simulink model "controller"  (R2020a)
settings: Solver=FixedStepDiscrete  StartTime=0.0  StopTime=10.0  FixedStep=0.01  MaxStep=0.01  RelTol=1e-3
undefined symbols (not defined in the file): DiscIntNeverNeededParam, PC_IST_den, PC_IST_num
libraries: simulink x10, dspsigattribs x1, dspfdesign x1
Description:
  | Ventilator Controller
settings Model: Creator=upattacini  LastModifiedBy=upattacini
settings SolverCC: MaxConsecutiveMinStep=10
settings DataIOCC: SaveOutput=off  SignalLogging=off  DSMLogging=off  SaveTime=off  ReturnWorkspaceOutputs=off
settings OptimizationCC: DefaultUnderspecifiedDataType=single  StrengthReduction=on  ZeroExternalMemoryAtStartup=off  ZeroInternalMemoryAtStartup=off  OptimizeBlockOrder=speed  OptimizationPriority=Speed  OptimizationCustomize=off  MultiThreadedLoops=on  EfficientTunableParamExpr=on
settings DebuggingCC: ParameterTunabilityLossMsg=error
settings SFSimCC: MATLABDynamicMemAlloc=off
settings RTWCC: SystemTargetFile=ert.tlc  GenCodeOnly=on  PackageGeneratedCodeAndArtifacts=on  PackageName=controller  TemplateMakefile=ert_default_tmf  TargetLang=C++
settings CodeAppCC: ForceParamTrailComments=on  IgnoreCustomStorageClasses=off  OperatorAnnotations=on  SimulinkDataObjDesc=on  SFDataObjDesc=on  InsertBlockDesc=on
settings ERTTargetCC: TargetLangStandard=C++03 (ISO)  GenerateSampleERTMain=on  MultiInstanceERTCode=on  CodeInterfacePackaging=C++ class  RootIOFormat=Structure reference  ERTCustomFileTemplate=example_file_process.tlc

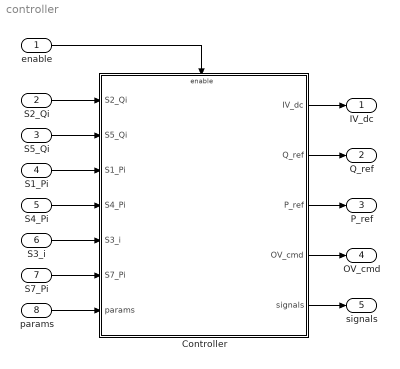
== system controller ==
  enable : Inport  OutDataTypeStr=boolean
  S2_Qi : Inport  Port=2  OutDataTypeStr=single
  S5_Qi : Inport  Port=3  OutDataTypeStr=single
  S1_Pi : Inport  Port=4  OutDataTypeStr=single
  S4_Pi : Inport  Port=5  OutDataTypeStr=single
  S3_i : Inport  Port=6  OutDataTypeStr=single  PortDimensions=2
  S7_Pi : Inport  Port=7  OutDataTypeStr=single
  params : Inport  Port=8  OutDataTypeStr=single  PortDimensions=3
  Controller : Subsystem  Tag=PublishSubsystem  mask(Controller){control_mode=IDLE, tidal_volume=0.65, PIP=25, PIP_step_perc=75, PIP_rise_perc=70, respiratory_rate=10, IE_ratio=1/2, HSC_cutoff=25, recovery_thres=1, VC_P=0.2, VC_I=10, VC_P_rec=0.1, VC_I_rec=5, PC_FFW=30, PC_P=1, PC_I=40, PC_FFW_rec=30, PC_P_rec=0.05, PC_I_rec=10, enable_trigger=off, pressure_thres=3, flowby_target=3}
      mask prompts: control_mode "Control Mode"; tidal_volume "Tidal Volume (L)"; PIP "PIP (cmH2O)"; PIP_step_perc "PIP Step Percentage (%)"; PIP_rise_perc "PIP Rising Percentage (%)"; respiratory_rate "Respiratory Rate (breaths/min)"; IE_ratio "Inspiration to Expiration Ratio"; HSC_cutoff "HSC Cutoff Frequency (Hz)"; recovery_thres "Threshold (bar)"; VC_P "Proportional (%FS/SLPM)"; VC_I "Integral (%FS/(SLPM*s))"; VC_P_rec "Proportional (%FS/SLPM)"; VC_I_rec "Integral (%FS/(SLPM*s))"; PC_FFW "Feed-Forward (%FS)"; PC_P "Proportional (%FS/cmH2O)"; PC_I "Integral (%FS/(cmH2O*s))"; PC_FFW_rec "Feed-Forward (%FS)"; PC_P_rec "Proportional (%FS/cmH2O)"; PC_I_rec "Integral (%FS/(cmH2O*s))"; enable_trigger "Enable Triggering"; pressure_thres "Pressure Threshold (cmH2O)"; flowby_target "Target Flow (L/min)"
      mask help: The controller generates the input signals that controls the inspiratory flow and expiratory valve.
      mask init:
      | Ts = eval(get_param(gcs, 'FixedStep'));
      mask TypeOptions control_mode: IDLE | CPAP | VCV | PRVC
      mask Callback control_mode:
      | numparams = Simulink.Mask.get(gcb).numParameters;
      | enable = cell(1, numparams);
      | enable(:) = {'on'};
      | 
      | control_mode = get_param(gcb, 'control_mode');
      | if strcmpi(control_mode, 'CPAP')
      |     enable{2} = 'off';
      |     enable(6:7) = {'off'};
      |     enable(10:13) = {'off'};
      | elseif strcmpi(control_mode, 'VCV')
      |     enable(3:5) = {'off'};
      |     enable(14:19) = {'off'};
      | elseif strcmpi(control_mode, 'PRVC')
      |     enable{2} = 'off';
      |     enable(10:13) = {'off'};
      | else
      |     enable(2:end) = {'off'};
      |     enable{8} = 'on';
      | end
      | if strcmpi(control_mode, 'CPAP')
      |     enable(end-2:end) = {'off'};
      | end
      | set_param(gcb, 'MaskEnables', enable);
      mask DialogControl Container2 Prompt: Medical Parameters
      mask DialogControl Container3 Prompt: Controller Parameters
      mask DialogControl Container4 Prompt: Filtering
      mask DialogControl Container5 Prompt: Gain Scheduling
      mask DialogControl Container6 Prompt: Volume Control Ventilation
      mask DialogControl Container7 Prompt: Standard Operations
      mask DialogControl Container8 Prompt: Recovery Operations
      mask DialogControl Container9 Prompt: Pressure Regulated Volume Control
      mask DialogControl Container10 Prompt: Standard Operations
      mask DialogControl Container11 Prompt: Recovery Operations
      mask DialogControl Container12 Prompt: Advanced Options
      mask DialogControl Container13 Prompt: Assisted Ventilation
      mask DialogControl Container14 Prompt: Flow-by
  IV_dc : Outport
  Q_ref : Outport  Port=2
  P_ref : Outport  Port=3
  OV_cmd : Outport  Port=4
  signals : Outport  Port=5
  wires:
  S2_Qi/1 -> Controller/1(S2_Qi)
  Controller/1(IV_dc) -> IV_dc/1
  Controller/2(Q_ref) -> Q_ref/1
  Controller/4(OV_cmd) -> OV_cmd/1
  S1_Pi/1 -> Controller/3(S1_Pi)
  Controller/3(P_ref) -> P_ref/1
  Controller/5(signals) -> signals/1
  enable/1 -> Controller/Enable
  S5_Qi/1 -> Controller/2(S5_Qi)
  S4_Pi/1 -> Controller/4(S4_Pi)
  params/1 -> Controller/7(params)
  S3_i/1 -> Controller/5(S3_i)
  S7_Pi/1 -> Controller/6(S7_Pi)

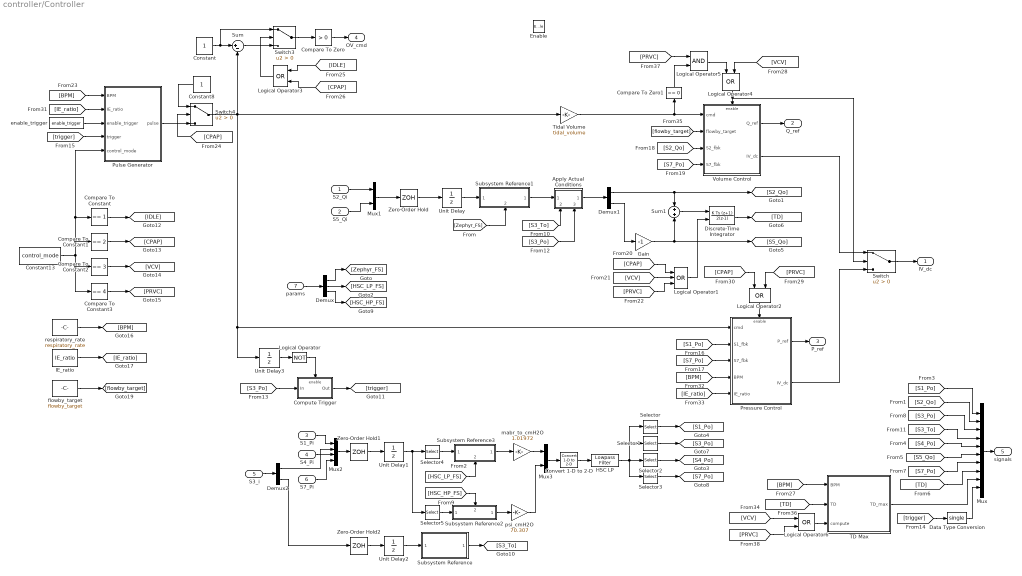
== system controller/Controller ==
  S2_Qi : Inport
  S5_Qi : Inport  Port=2
  S1_Pi : Inport  Port=3
  S4_Pi : Inport  Port=4
  S3_i : Inport  Port=5
  S7_Pi : Inport  Port=6
  params : Inport  Port=7
  Enable : EnablePort  StatesWhenEnabling=reset
  Apply Actual Conditions : Subsystem  ReferencedSubsystem=apply_actual_conditions
      settings: PortSchema="{\"entries\":[{\"content\":{\"sides\":[{\"content\":{\"connectorIds\":[\"In1\"]},\"type\":\"ConnectorPlacement.EquallySpacedRectSide\",\"uuid\":\"3b4e15f5-ec7a-455d-a112-e063b421ee9f\"},{\"content\":{\"connectorIds\":[\"Out1\"],\"side\":\"RIGHT\"},\"type\":\"ConnectorPlacement.EquallySpacedRectSide\",\"uuid\":\"595b3fd5-6603-4191-b183-4edf5336d9a2\"},{\"content\":{\"connectorIds\":[],\"side\":\"TOP\"},\"type\":\"ConnectorPlacement.EquallySpacedRectSide\",\"uuid\":\"7211f4ea-7225-4536-b1e6-5aea95971c19\"},{\"content\":{\"connectorIds\":[\"In2\",\"In3\"],\"side\":\"BOTTOM\"},\"type\":\"ConnectorPlacement.EquallySpacedRectSide\",\"uuid\":\"c060314b-2654-4a54-a68c-60767f6efbb5\"}]},\"type\":\"ConnectorPlacement.EquallySpacedConnector\",\"uuid\":\"0e2934c3-16fd-4aed-85e0-c12757e58969\"}],\"packageUris\":[\"http://schema.mathworks.com/mf0/Connector/19700101\"],\"version\":\"1.0\"}"
  Compare To Constant : simulink/Logic and Bit Operations/Compare To Constant  relop===  const=1  OutDataTypeStr=boolean
  Compare To Constant1 : simulink/Logic and Bit Operations/Compare To Constant  relop===  const=2  OutDataTypeStr=boolean
  Compare To Constant2 : simulink/Logic and Bit Operations/Compare To Constant  relop===  const=3  OutDataTypeStr=boolean
  Compare To Constant3 : simulink/Logic and Bit Operations/Compare To Constant  relop===  const=4  OutDataTypeStr=boolean
  Compare To Zero : simulink/Logic and Bit Operations/Compare To Zero  relop=>  OutDataTypeStr=boolean
  Compare To Zero1 : simulink/Logic and Bit Operations/Compare To Zero  relop===  OutDataTypeStr=boolean
  Compute Trigger : Subsystem
  Constant : Constant  OutDataTypeStr=single
  Constant13 : Constant  Value=control_mode  OutDataTypeStr=uint8
  Constant8 : Constant  OutDataTypeStr=single
  Convert 1-D to 2-D : dspsigattribs/Convert 1-D to 2-D  M=1  N=4  frameBasedOut=off
      settings: SourceProductBaseCode=DS
  Data Type Conversion : DataTypeConversion  OutDataTypeStr=single
  Demux : Demux  Outputs=3
  Demux1 : Demux  Outputs=2
  Demux2 : Demux  Outputs=2
  Discrete-Time Integrator : DiscreteIntegrator  IntegratorMethod=Integration: Trapezoidal  gainval=1/60  ExternalReset=rising  SampleTime=-1  ICPrevOutput=DiscIntNeverNeededParam  ICPrevScaledInput=DiscIntNeverNeededParam
  Gain : Gain  Gain=-1
  HSC LP : dspfdesign/Lowpass Filter  FilterType=IIR  DesignForMinimumOrder=off  FilterOrder=3  PassbandFrequency=HSC_cutoff  StopbandFrequency=12e3  PassbandRipple=0.5  StopbandAttenuation=30  InheritSampleRate=on  SampleRate=44100  SimulateUsing=Code generation  roundingMode=Floor  coeffsDataTypeStr=fixdt(1,16)
  IE_ratio : Constant  Value=IE_ratio  OutDataTypeStr=single
  Logical Operator : Logic  Operator=NOT  AllPortsSameDT=off  OutDataTypeStr=boolean
  Logical Operator1 : Logic  Operator=OR  Inputs=3  AllPortsSameDT=off  OutDataTypeStr=boolean
  Logical Operator{2..4,6} (4 alike) : Logic  Operator=OR  AllPortsSameDT=off  OutDataTypeStr=boolean
  Logical Operator5 : Logic  AllPortsSameDT=off  OutDataTypeStr=boolean
  Mux : Mux  Inputs=10
  Mux1 : Mux  Inputs=2
  Mux2 : Mux
  Mux3 : Mux  Inputs=2
  Pressure Control : Subsystem
  Pulse Generator : Stateflow chart  TreatAsAtomicUnit=on
      settings: PortSchema="{\"entries\":[{\"content\":{\"sides\":[{\"content\":{\"connectorIds\":[\"In1\",\"In2\",\"In4\",\"In5\",\"In3\"]},\"type\":\"ConnectorPlacement.EquallySpacedRectSide\",\"uuid\":\"cac98c0d-34b3-4e58-8046-b8c4efc2c89e\"},{\"content\":{\"connectorIds\":[\"Out1\"],\"side\":\"RIGHT\"},\"type\":\"ConnectorPlacement.EquallySpacedRectSide\",\"uuid\":\"54f456d4-4e16-46b8-85c9-ac589a430e9a\"},{\"content\":{\"connectorIds\":[],\"side\":\"TOP\"},\"type\":\"ConnectorPlacement.EquallySpacedRectSide\",\"uuid\":\"89fc85cb-8402-4155-a34e-39605e1a4b07\"}]},\"type\":\"ConnectorPlacement.EquallySpacedConnector\",\"uuid\":\"7c549002-3361-42b3-b309-390e5b6446c3\"}],\"packageUris\":[\"http://schema.mathworks.com/mf0/Connector/19700101\"],\"version\":\"1.0\"}"
  Selector : Selector  InputPortWidth=4  IndexOptions=Index vector (dialog)  Indices=1  OutputSizes=1
  Selector1 : Selector  InputPortWidth=4  IndexOptions=Index vector (dialog)  Indices=2  OutputSizes=1
  Selector2 : Selector  InputPortWidth=4  IndexOptions=Index vector (dialog)  Indices=3  OutputSizes=1
  Selector3 : Selector  InputPortWidth=4  IndexOptions=Index vector (dialog)  Indices=4  OutputSizes=1
  Selector4 : Selector  InputPortWidth=4  IndexOptions=Index vector (dialog)  Indices=[1 2 3]  OutputSizes=1
  Selector5 : Selector  InputPortWidth=4  IndexOptions=Index vector (dialog)  Indices=4  OutputSizes=1
  Subsystem Reference : Subsystem  ReferencedSubsystem=temperature_decoder
  Subsystem Reference1 : Subsystem  ReferencedSubsystem=absolute_decoder
      settings: PortSchema="{\"entries\":[{\"content\":{\"sides\":[{\"content\":{\"connectorIds\":[\"In1\"]},\"type\":\"ConnectorPlacement.EquallySpacedRectSide\",\"uuid\":\"2ef0a3f0-f31e-4d03-a173-55859c118317\"},{\"content\":{\"connectorIds\":[\"Out1\"],\"side\":\"RIGHT\"},\"type\":\"ConnectorPlacement.EquallySpacedRectSide\",\"uuid\":\"777c94e1-db74-470f-8997-0780b50ff5fd\"},{\"content\":{\"connectorIds\":[],\"side\":\"TOP\"},\"type\":\"ConnectorPlacement.EquallySpacedRectSide\",\"uuid\":\"3869b089-f921-4789-b3c4-768f35a800e8\"},{\"content\":{\"connectorIds\":[\"In2\"],\"side\":\"BOTTOM\"},\"type\":\"ConnectorPlacement.EquallySpacedRectSide\",\"uuid\":\"61a1bb3c-7da2-4a2b-ab0e-5315ec9e9a55\"}]},\"type\":\"ConnectorPlacement.EquallySpacedConnector\",\"uuid\":\"f5d8d852-93e3-4839-9332-278801ab0ff2\"}],\"packageUris\":[\"http://schema.mathworks.com/mf0/Connector/19700101\"],\"version\":\"1.0\"}"
  Subsystem Reference2 : Subsystem  ReferencedSubsystem=absolute_decoder
      settings: PortSchema="{\"entries\":[{\"content\":{\"sides\":[{\"content\":{\"connectorIds\":[\"In1\"]},\"type\":\"ConnectorPlacement.EquallySpacedRectSide\",\"uuid\":\"2ef0a3f0-f31e-4d03-a173-55859c118317\"},{\"content\":{\"connectorIds\":[\"Out1\"],\"side\":\"RIGHT\"},\"type\":\"ConnectorPlacement.EquallySpacedRectSide\",\"uuid\":\"777c94e1-db74-470f-8997-0780b50ff5fd\"},{\"content\":{\"connectorIds\":[\"In2\"],\"side\":\"TOP\"},\"type\":\"ConnectorPlacement.EquallySpacedRectSide\",\"uuid\":\"3869b089-f921-4789-b3c4-768f35a800e8\"}]},\"type\":\"ConnectorPlacement.EquallySpacedConnector\",\"uuid\":\"f5d8d852-93e3-4839-9332-278801ab0ff2\"}],\"packageUris\":[\"http://schema.mathworks.com/mf0/Connector/19700101\"],\"version\":\"1.0\"}"
  Subsystem Reference3 : Subsystem  ReferencedSubsystem=differential_decoder
      settings: PortSchema="{\"entries\":[{\"content\":{\"sides\":[{\"content\":{\"connectorIds\":[\"In1\"]},\"type\":\"ConnectorPlacement.EquallySpacedRectSide\",\"uuid\":\"2ef0a3f0-f31e-4d03-a173-55859c118317\"},{\"content\":{\"connectorIds\":[\"Out1\"],\"side\":\"RIGHT\"},\"type\":\"ConnectorPlacement.EquallySpacedRectSide\",\"uuid\":\"777c94e1-db74-470f-8997-0780b50ff5fd\"},{\"content\":{\"connectorIds\":[],\"side\":\"TOP\"},\"type\":\"ConnectorPlacement.EquallySpacedRectSide\",\"uuid\":\"3869b089-f921-4789-b3c4-768f35a800e8\"},{\"content\":{\"connectorIds\":[\"In2\"],\"side\":\"BOTTOM\"},\"type\":\"ConnectorPlacement.EquallySpacedRectSide\",\"uuid\":\"b0751dc2-7c78-44d3-b598-d7c6b3cf40a8\"}]},\"type\":\"ConnectorPlacement.EquallySpacedConnector\",\"uuid\":\"f5d8d852-93e3-4839-9332-278801ab0ff2\"}],\"packageUris\":[\"http://schema.mathworks.com/mf0/Connector/19700101\"],\"version\":\"1.0\"}"
  Sum : Sum  Inputs=|+-
  Sum1 : Sum
  Switch : Switch  Criteria=u2 > Threshold
  Switch3 : Switch  Criteria=u2 > Threshold  OutDataTypeStr=single
  Switch4 : Switch  Criteria=u2 > Threshold  OutDataTypeStr=single
  TD Max : Stateflow chart  TreatAsAtomicUnit=on
      settings: PortSchema="{\"entries\":[{\"content\":{\"sides\":[{\"content\":{\"connectorIds\":[\"In1\",\"In3\",\"In2\"]},\"type\":\"ConnectorPlacement.EquallySpacedRectSide\",\"uuid\":\"fecf34d5-cdf1-464c-9ca9-d83d0877460d\"},{\"content\":{\"connectorIds\":[\"Out1\"],\"side\":\"RIGHT\"},\"type\":\"ConnectorPlacement.EquallySpacedRectSide\",\"uuid\":\"3cbf9760-b18e-491c-a2ff-c2213a779b1e\"},{\"content\":{\"connectorIds\":[],\"side\":\"TOP\"},\"type\":\"ConnectorPlacement.EquallySpacedRectSide\",\"uuid\":\"225e4322-780b-497a-9f73-62f2fd006c1b\"}]},\"type\":\"ConnectorPlacement.EquallySpacedConnector\",\"uuid\":\"c002febf-6ffa-4c13-b9a0-228d22517978\"}],\"packageUris\":[\"http://schema.mathworks.com/mf0/Connector/19700101\"],\"version\":\"1.0\"}"
  Tidal Volume : Gain  Gain=tidal_volume
  Unit Delay : UnitDelay  SampleTime=-1  HasFrameUpgradeWarning=on
  Unit Delay1 : UnitDelay  InitialCondition=2^14 * [0.5 0.5 0.5 0]  SampleTime=-1  HasFrameUpgradeWarning=on
  Unit Delay2 : UnitDelay  SampleTime=-1  HasFrameUpgradeWarning=on
  Unit Delay3 : UnitDelay  SampleTime=-1  HasFrameUpgradeWarning=on
  Volume Control : Subsystem
  Zero-Order Hold : ZeroOrderHold  SampleTime=Ts
  Zero-Order Hold1 : ZeroOrderHold  SampleTime=Ts
  Zero-Order Hold2 : ZeroOrderHold  SampleTime=Ts
  enable_trigger : Constant  Value=enable_trigger  OutDataTypeStr=boolean
  flowby_target : Constant  Value=flowby_target  OutDataTypeStr=single
  mabr_to_cmH2O : Gain  Gain=1.01972
  psi_cmH2O : Gain  Gain=70.307
  respiratory_rate : Constant  Value=respiratory_rate  OutDataTypeStr=single
  IV_dc : Outport  OutputWhenDisabled=reset  InitialOutput=0
  Q_ref : Outport  Port=2  OutputWhenDisabled=reset  InitialOutput=0
  P_ref : Outport  Port=3  OutputWhenDisabled=reset  InitialOutput=0
  OV_cmd : Outport  Port=4  OutputWhenDisabled=reset  InitialOutput=0
  signals : Outport  Port=5  OutputWhenDisabled=reset  InitialOutput=0
  wires:
  Constant/1 -> Switch3/1, Sum/1
  Volume Control/1(Q_ref) -> Q_ref/1
  Switch/1 -> IV_dc/1
  Volume Control/2(IV_dc) -> Switch/1
  Pressure Control/2(IV_dc) -> Switch/3
  Pressure Control/1(P_ref) -> P_ref/1
  params/1 -> Demux/1
  Demux/1 -> [Zephyr_FS]
  [Zephyr_FS] -> Subsystem Reference1/2
  Mux/1 -> signals/1
  Zero-Order Hold/1 -> Unit Delay/1
  Zero-Order Hold1/1 -> Unit Delay1/1
  Unit Delay1/1 -> Selector5/1, Selector4/1
  Demux/2 -> [HSC_LP_FS]
  Gain/1 -> Sum1/2, [S5_Qo]
  Discrete-Time Integrator/1 -> [TD]
  S2_Qi/1 -> Mux1/1
  S5_Qi/1 -> Mux1/2
  Mux1/1 -> Zero-Order Hold/1
  Mux2/1 -> Zero-Order Hold1/1
  Convert 1-D to 2-D/1 -> HSC LP/1
  HSC LP/1 -> Selector/1, Selector1/1, Selector3/1, Selector2/1
  S7_Pi/1 -> Mux2/4
  Selector3/1 -> [S7_Po]
  Demux/3 -> [HSC_HP_FS]
  Selector4/1 -> Subsystem Reference3/1
  Selector5/1 -> Subsystem Reference2/1
  Subsystem Reference3/1 -> mabr_to_cmH2O/1
  Subsystem Reference2/1 -> psi_cmH2O/1
  S1_Pi/1 -> Mux2/1
  Demux2/2 -> Zero-Order Hold2/1
  S3_i/1 -> Demux2/1
  Demux1/1 -> Sum1/1, [S2_Qo]
  Demux1/2 -> Gain/1
  Unit Delay2/1 -> Subsystem Reference/1
  Zero-Order Hold2/1 -> Unit Delay2/1
  Subsystem Reference/1 -> [S3_To]
  [S3_To] -> Apply Actual Conditions/2
  Unit Delay/1 -> Subsystem Reference1/1
  Subsystem Reference1/1 -> Apply Actual Conditions/1
  Apply Actual Conditions/1 -> Demux1/1
  Sum1/1 -> Discrete-Time Integrator/1
  Compute Trigger/1(Out) -> [trigger]
  Switch4/1 -> Unit Delay3/1, Pressure Control/1(cmd), Tidal Volume/1, Sum/2
  Logical Operator/1 -> Compute Trigger/Enable
  [S3_Po] -> Apply Actual Conditions/3
  Mux3/1 -> Convert 1-D to 2-D/1
  Logical Operator2/1 -> Pressure Control/Enable
  [PRVC] -> Logical Operator2/2
  Switch3/1 -> Compare To Zero/1
  Sum/1 -> Switch3/3
  [CPAP] -> Switch4/2
  Constant8/1 -> Switch4/1
  Logical Operator3/1 -> Switch3/2
  [IDLE] -> Logical Operator3/1
  [CPAP] -> Logical Operator3/2
  Unit Delay3/1 -> Logical Operator/1
  [S3_Po] -> Compute Trigger/1(In)
  Selector/1 -> [S1_Po]
  [S1_Po] -> Pressure Control/2(S1_fbk)
  [S7_Po] -> Pressure Control/3(S7_fbk)
  [S2_Qo] -> Volume Control/3(S2_fbk)
  [S7_Po] -> Volume Control/4(S7_fbk)
  Compare To Zero/1 -> OV_cmd/1
  [S3_To] -> Mux/4
  [S4_Po] -> Mux/5
  [S3_Po] -> Mux/3
  [S5_Qo] -> Mux/6
  [S2_Qo] -> Mux/2
  [S7_Po] -> Mux/7
  [S1_Po] -> Mux/1
  [TD] -> Mux/8
  [trigger] -> Data Type Conversion/1
  [VCV] -> Logical Operator1/2
  [CPAP] -> Logical Operator1/1
  [PRVC] -> Logical Operator1/3
  Logical Operator1/1 -> Discrete-Time Integrator/2
  Compare To Constant/1 -> [IDLE]
  Compare To Constant1/1 -> [CPAP]
  Compare To Constant2/1 -> [VCV]
  Compare To Constant3/1 -> [PRVC]
  [CPAP] -> Logical Operator2/1
  [HSC_LP_FS] -> Subsystem Reference3/2
  [HSC_HP_FS] -> Subsystem Reference2/2
  mabr_to_cmH2O/1 -> Mux3/1
  psi_cmH2O/1 -> Mux3/2
  Demux2/1 -> Mux2/2
  S4_Pi/1 -> Mux2/3
  Selector1/1 -> [S3_Po]
  Selector2/1 -> [S4_Po]
  Tidal Volume/1 -> Compare To Zero1/1, Volume Control/1(cmd)
  respiratory_rate/1 -> [BPM]
  IE_ratio/1 -> [IE_ratio]
  [BPM] -> Pulse Generator/1(BPM)
  [IE_ratio] -> Pulse Generator/2(IE_ratio)
  [BPM] -> Pressure Control/4(BPM)
  [IE_ratio] -> Pressure Control/5(IE_ratio)
  Constant13/1 -> Compare To Constant1/1, Compare To Constant/1, Pulse Generator/3(control_mode), Compare To Constant2/1, Compare To Constant3/1
  enable_trigger/1 -> Pulse Generator/4(enable_trigger)
  [trigger] -> Pulse Generator/5(trigger)
  Pulse Generator/1(pulse) -> Switch4/3
  flowby_target/1 -> [flowby_target]
  [flowby_target] -> Volume Control/2(flowby_target)
  Logical Operator4/1 -> Switch/2, Volume Control/Enable
  [VCV] -> Logical Operator4/2
  Logical Operator5/1 -> Logical Operator4/1
  [PRVC] -> Logical Operator5/1
  Compare To Zero1/1 -> Logical Operator5/2
  [BPM] -> TD Max/1(BPM)
  [TD] -> TD Max/3(TD)
  Logical Operator6/1 -> TD Max/2(compute)
  [VCV] -> Logical Operator6/1
  [PRVC] -> Logical Operator6/2
  TD Max/1(TD_max) -> Mux/9
  Data Type Conversion/1 -> Mux/10

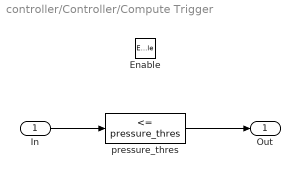
== system controller/Controller/Compute Trigger ==
  In : Inport
  Enable : EnablePort  StatesWhenEnabling=reset
  pressure_thres : simulink/Logic and Bit Operations/Compare To Constant  relop=<=  const=pressure_thres  OutDataTypeStr=boolean
  Out : Outport  OutputWhenDisabled=reset  InitialOutput=0
  wires:
  In/1 -> pressure_thres/1
  pressure_thres/1 -> Out/1

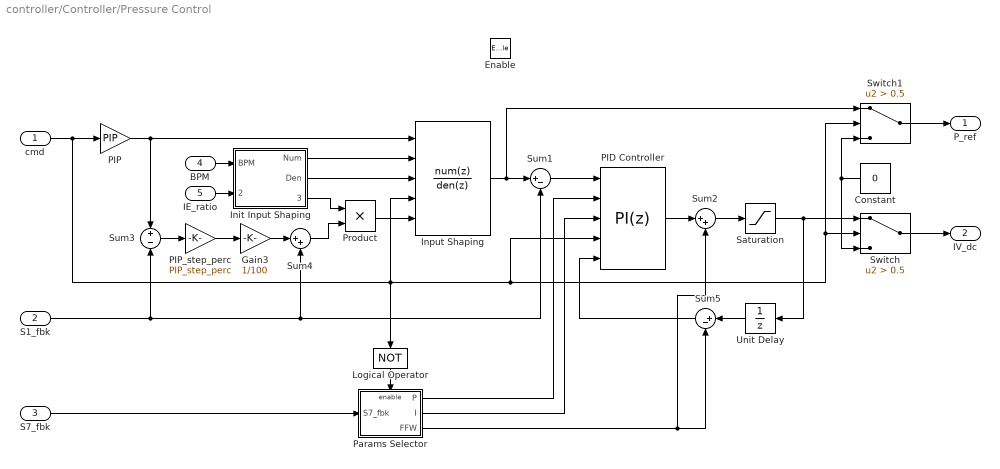
== system controller/Controller/Pressure Control ==
  cmd : Inport
  S1_fbk : Inport  Port=2
  S7_fbk : Inport  Port=3
  BPM : Inport  Port=4
  IE_ratio : Inport  Port=5
  Enable : EnablePort  StatesWhenEnabling=reset
  Constant : Constant  Value=0  OutDataTypeStr=single
  Gain3 : Gain  Gain=1/100
  Init Input Shaping : Subsystem
  Input Shaping : DiscreteFilter  NumeratorSource=Input port  Numerator=PC_IST_num  DenominatorSource=Input port  Denominator=PC_IST_den  InitialStatesSource=Input port  ExternalReset=Rising  a0EqualsOne=on
      settings: InputPortMap=u0,p1,p3,r7,p5
  Logical Operator : Logic  Operator=NOT  AllPortsSameDT=off  OutDataTypeStr=boolean
  PID Controller : simulink/Continuous/PID Controller  Controller=PI  Form=Parallel  TimeDomain=Discrete-time  UseExternalTs=off  SampleTime=-1  IntegratorMethod=Trapezoidal  FilterMethod=Trapezoidal  ControllerParametersSource=external  P=PC_P  I=PC_I  D=1  UseFilter=on  N=100  TunerSelectOption=Transfer Function Based (PID Tuner App)  InitialConditionSource=internal  InitialConditionForIntegrator=0  InitialConditionForFilter=0  DifferentiatorICPrevScaledInput=0  ExternalReset=rising  TrackingMode=on  Kt=1  LimitOutput=off  UpperSaturationLimit=100  LowerSaturationLimit=0  LinearizeAsGain=on  AntiWindupMode=clamping  Kb=1  POutMin=[]  POutMax=[]  IOutMin=[]  IOutMax=[]  DOutMin=[]  DOutMax=[]  NOutMin=[]  NOutMax=[]  SumOutMin=[]  SumOutMax=[]  SaturationOutMin=[]  SaturationOutMax=[]  PParamMin=[]  PParamMax=[]  IParamMin=[]  IParamMax=[]  DParamMin=[]  DParamMax=[]  NParamMin=[]  NParamMax=[]  KbParamMin=[]  KbParamMax=[]  KtParamMin=[]  KtParamMax=[]  KbOutMin=[]  KbOutMax=[]  KtOutMin=[]  KtOutMax=[]  IntegratorOutMin=[]  IntegratorOutMax=[]  FilterOutMin=[]  FilterOutMax=[]  SumI1OutMin=[]  SumI1OutMax=[]  SumI2OutMin=[]  SumI2OutMax=[]  SumI3OutMin=[]  SumI3OutMax=[]  SumI4OutMin=[]  SumI4OutMax=[]  SumDOutMin=[]  SumDOutMax=[]  DifferentiatorOutMin=[]  DifferentiatorOutMax=[]  FilterDiffOutCoefMin=[]  FilterDiffOutCoefMax=[]  ReciprocalOutMin=[]  ReciprocalOutMax=[]  SumDenOutMin=[]  SumDenOutMax=[]  SumNumOutMin=[]  SumNumOutMax=[]  DivideOutMin=[]  DivideOutMax=[]  UdiffTsProdOutMin=[]  UdiffTsProdOutMax=[]  NTsProdOutMin=[]  NTsProdOutMax=[]  UintegralTsProdOutMin=[]  UintegralTsProdOutMax=[]  UngainTsProdOutMin=[]  UngainTsProdOutMax=[]  IntegratorContinuousStateAttributes=''  IntegratorStateMustResolveToSignalObject=off  IntegratorRTWStateStorageClass=Auto  FilterContinuousStateAttributes=''  FilterStateMustResolveToSignalObject=off  FilterRTWStateStorageClass=Auto  ParallelPVariant=ExternalParameters  IdealPVariant=Disabled  IVariant=ExternalParameters  DVariant=Disabled  IntegratorVariant=Discrete  SatVariant=Disabled  AWVariant=Passthrough  PCopyVariant=Disabled  TRVariant=Enabled  FdbkBlocksVariant=Feedback  IdealPFdbkVariant=Passthrough  SatFdbkVariant=Passthrough  DerivativeFilterVariant=Disabled  NVariant=Disabled  NCopyVariant=Disabled_SignalSpec  FilterICVariant=Disabled  IntegratorICVariant=InternalICs  ExternalResetVariant=ExternalReset  TRSumVariant=TrackingMode  SumFdbkVariant=Enabled  SumVariant=Sum_PI  TsampFilterVariant=InternalTs  TsampNgainVariant=Passthrough  TsampIntegralVariant=Passthrough
  PIP : Gain  Gain=PIP
  PIP_step_perc : Gain  Gain=PIP_step_perc
  Params Selector : Subsystem
  Product : Product
  Saturation : Saturate  UpperLimit=100  LowerLimit=0
  Sum1 : Sum  Inputs=|+-
  Sum2 : Sum  Inputs=|++
  Sum3 : Sum  Inputs=+-
  Sum4 : Sum  Inputs=|++
  Sum5 : Sum  Inputs=|+-
  Switch : Switch  Criteria=u2 > Threshold  Threshold=0.5
  Switch1 : Switch  Criteria=u2 > Threshold  Threshold=0.5
  Unit Delay : UnitDelay  SampleTime=-1  HasFrameUpgradeWarning=on
  P_ref : Outport  OutputWhenDisabled=reset  InitialOutput=0
  IV_dc : Outport  Port=2  OutputWhenDisabled=reset  InitialOutput=0
  wires:
  Sum1/1 -> PID Controller/1
  Saturation/1 -> Switch/1, Unit Delay/1
  Switch/1 -> IV_dc/1
  Switch1/1 -> P_ref/1
  PIP/1 -> Input Shaping/1, Sum3/1
  S1_fbk/1 -> Sum1/2, Sum4/2, Sum3/2
  cmd/1 -> PIP/1, Switch1/2, Switch/2, PID Controller/4, Input Shaping/4, Logical Operator/1
  Input Shaping/1 -> Switch1/1, Sum1/1
  Sum3/1 -> PIP_step_perc/1
  Product/1 -> Input Shaping/5
  PIP_step_perc/1 -> Gain3/1
  Constant/1 -> Switch1/3, Switch/3
  S7_fbk/1 -> Params Selector/1(S7_fbk)
  PID Controller/1 -> Sum2/1
  Sum2/1 -> Saturation/1
  Params Selector/3(FFW) -> Sum5/2, Sum2/2
  Unit Delay/1 -> Sum5/1
  Sum5/1 -> PID Controller/5
  Logical Operator/1 -> Params Selector/Enable
  Params Selector/1(P) -> PID Controller/2
  Params Selector/2(I) -> PID Controller/3
  Gain3/1 -> Sum4/1
  Init Input Shaping/1(Num) -> Input Shaping/2
  Init Input Shaping/2(Den) -> Input Shaping/3
  Init Input Shaping/3(x0_Gain) -> Product/1
  Sum4/1 -> Product/2
  BPM/1 -> Init Input Shaping/1(BPM)
  IE_ratio/1 -> Init Input Shaping/2(IE_ratio)

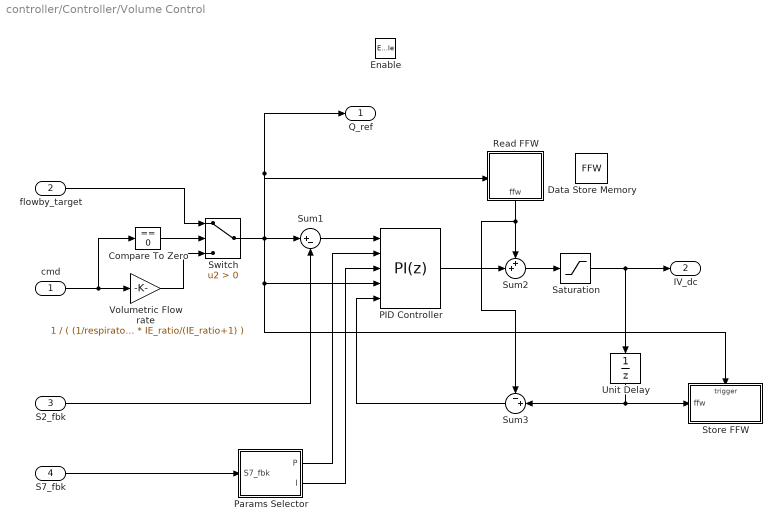
== system controller/Controller/Volume Control ==
  cmd : Inport
  flowby_target : Inport  Port=2
  S2_fbk : Inport  Port=3
  S7_fbk : Inport  Port=4
  Enable : EnablePort
  Compare To Zero : simulink/Logic and Bit Operations/Compare To Zero  relop===  OutDataTypeStr=boolean
  Data Store Memory : DataStoreMemory  DataStoreName=FFW  ReadBeforeWriteMsg=warning  WriteAfterWriteMsg=warning  WriteAfterReadMsg=warning  ShowAdditionalParam=off  OutMin=0  OutMax=100
  PID Controller : simulink/Continuous/PID Controller  Controller=PI  Form=Parallel  TimeDomain=Discrete-time  UseExternalTs=off  SampleTime=-1  IntegratorMethod=Trapezoidal  FilterMethod=Forward Euler  ControllerParametersSource=external  P=VC_P  I=VC_I  D=1  UseFilter=on  N=100  TunerSelectOption=Transfer Function Based (PID Tuner App)  InitialConditionSource=internal  InitialConditionForIntegrator=0  InitialConditionForFilter=0  DifferentiatorICPrevScaledInput=0  ExternalReset=either  TrackingMode=on  Kt=1  LimitOutput=off  UpperSaturationLimit=100  LowerSaturationLimit=0  LinearizeAsGain=on  AntiWindupMode=clamping  Kb=1  POutMin=[]  POutMax=[]  IOutMin=[]  IOutMax=[]  DOutMin=[]  DOutMax=[]  NOutMin=[]  NOutMax=[]  SumOutMin=[]  SumOutMax=[]  SaturationOutMin=[]  SaturationOutMax=[]  PParamMin=[]  PParamMax=[]  IParamMin=[]  IParamMax=[]  DParamMin=[]  DParamMax=[]  NParamMin=[]  NParamMax=[]  KbParamMin=[]  KbParamMax=[]  KtParamMin=[]  KtParamMax=[]  KbOutMin=[]  KbOutMax=[]  KtOutMin=[]  KtOutMax=[]  IntegratorOutMin=[]  IntegratorOutMax=[]  FilterOutMin=[]  FilterOutMax=[]  SumI1OutMin=[]  SumI1OutMax=[]  SumI2OutMin=[]  SumI2OutMax=[]  SumI3OutMin=[]  SumI3OutMax=[]  SumI4OutMin=[]  SumI4OutMax=[]  SumDOutMin=[]  SumDOutMax=[]  DifferentiatorOutMin=[]  DifferentiatorOutMax=[]  FilterDiffOutCoefMin=[]  FilterDiffOutCoefMax=[]  ReciprocalOutMin=[]  ReciprocalOutMax=[]  SumDenOutMin=[]  SumDenOutMax=[]  SumNumOutMin=[]  SumNumOutMax=[]  DivideOutMin=[]  DivideOutMax=[]  UdiffTsProdOutMin=[]  UdiffTsProdOutMax=[]  NTsProdOutMin=[]  NTsProdOutMax=[]  UintegralTsProdOutMin=[]  UintegralTsProdOutMax=[]  UngainTsProdOutMin=[]  UngainTsProdOutMax=[]  IntegratorContinuousStateAttributes=''  IntegratorStateMustResolveToSignalObject=off  IntegratorRTWStateStorageClass=Auto  FilterContinuousStateAttributes=''  FilterStateMustResolveToSignalObject=off  FilterRTWStateStorageClass=Auto  ParallelPVariant=ExternalParameters  IdealPVariant=Disabled  IVariant=ExternalParameters  DVariant=Disabled  IntegratorVariant=Discrete  SatVariant=Disabled  AWVariant=Passthrough  PCopyVariant=Disabled  TRVariant=Enabled  FdbkBlocksVariant=Feedback  IdealPFdbkVariant=Passthrough  SatFdbkVariant=Passthrough  DerivativeFilterVariant=Disabled  NVariant=Disabled  NCopyVariant=Disabled_SignalSpec  FilterICVariant=Disabled  IntegratorICVariant=InternalICs  ExternalResetVariant=ExternalReset  TRSumVariant=TrackingMode  SumFdbkVariant=Enabled  SumVariant=Sum_PI  TsampFilterVariant=InternalTs  TsampNgainVariant=Passthrough  TsampIntegralVariant=Passthrough
  Params Selector : Subsystem
  Read FFW : Subsystem  TreatAsAtomicUnit=on
  Saturation : Saturate  UpperLimit=100  LowerLimit=0
  Store FFW : Subsystem  TreatAsAtomicUnit=on
  Sum1 : Sum  Inputs=|+-
  Sum2 : Sum  Inputs=++|
  Sum3 : Sum  Inputs=-+|
  Switch : Switch  Criteria=u2 > Threshold
  Unit Delay : UnitDelay  SampleTime=-1  HasFrameUpgradeWarning=on
  Volumetric Flow rate : Gain  Gain=1 / ( (1/respiratory_rate) * IE_ratio/(IE_ratio+1) )
  Q_ref : Outport  OutputWhenDisabled=reset  InitialOutput=0
  IV_dc : Outport  Port=2  OutputWhenDisabled=reset  InitialOutput=0
  wires:
  Read FFW/1(ffw) -> Sum3/1, Sum2/1
  Switch/1 -> Q_ref/1, Read FFW/Enable, Store FFW/Trigger, PID Controller/4, Sum1/1
  cmd/1 -> Compare To Zero/1, Volumetric Flow rate/1
  Sum2/1 -> Saturation/1
  Sum1/1 -> PID Controller/1
  PID Controller/1 -> Sum2/2
  Saturation/1 -> IV_dc/1, Unit Delay/1
  S2_fbk/1 -> Sum1/2
  Sum3/1 -> PID Controller/5
  Unit Delay/1 -> Store FFW/1(ffw), Sum3/2
  S7_fbk/1 -> Params Selector/1(S7_fbk)
  Params Selector/1(P) -> PID Controller/2
  Params Selector/2(I) -> PID Controller/3
  Volumetric Flow rate/1 -> Switch/3
  flowby_target/1 -> Switch/1
  Compare To Zero/1 -> Switch/2

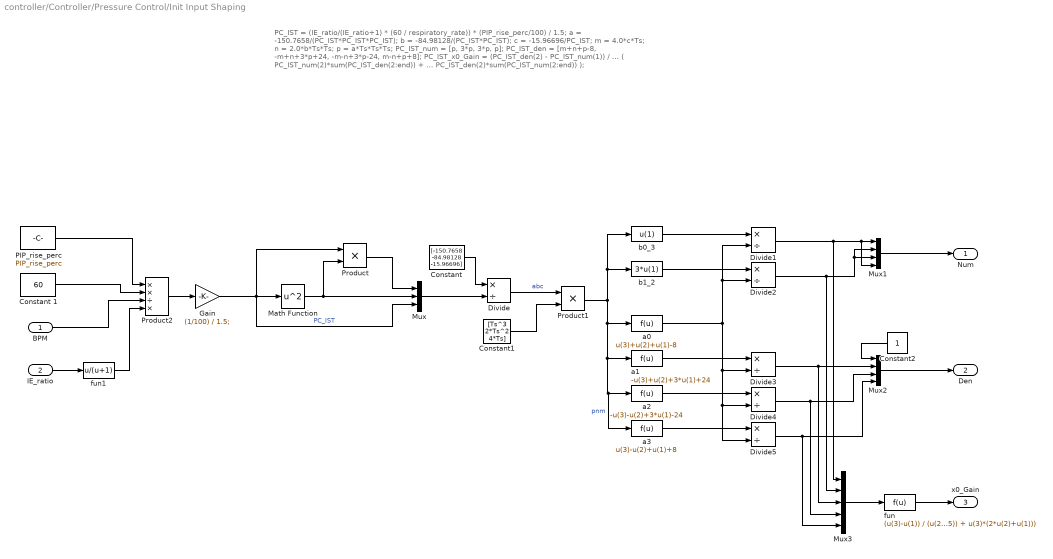
== system controller/Controller/Pressure Control/Init Input Shaping ==
  note: PC_IST = (IE_ratio/(IE_ratio+1) * (60 / respiratory_rate)) * (PIP_rise_perc/100) / 1.5;
      | a = -150.7658/(PC_IST*PC_IST*PC_IST);
      | b = -84.98128/(PC_IST*PC_IST);
      | c = -15.96696/PC_IST;
      |
      | m = 4.0*c*Ts;
      | n = 2.0*b*Ts*Ts;
      | p = a*Ts*Ts*Ts;
      |
      | PC_IST_num = [p, 3*p, 3*p, p];
      | PC_IST_den = [m+n+p-8, -m+n+3*p+24, -m-n+3*p-24, m-n+p+8];
      | PC_IST_x0_Gain = (PC_IST_den(2) - PC_IST_num(1)) / ...
      |                                 ( PC_IST_num(2)*sum(PC_IST_den(2:end)) + ...
      |                                  PC_IST_den(2)*sum(PC_IST_num(2:end)) );
  BPM : Inport
  IE_ratio : Inport  Port=2
  Constant : Constant  Value=[-150.7658 -84.98128 -15.96696]  OutDataTypeStr=single
  Constant 1 : Constant  Value=60  OutDataTypeStr=single
  Constant1 : Constant  Value=[Ts^3 2*Ts^2 4*Ts]  OutDataTypeStr=single
  Constant2 : Constant  OutDataTypeStr=single
  Divide{,1..5} (6 alike) : Product  Inputs=*/
  Gain : Gain  Gain=(1/100) / 1.5;
  Math Function : Math  Operator=square  SaturateOnIntegerOverflow=on
  Mux : Mux  Inputs=3
  Mux1 : Mux
  Mux2 : Mux
  Mux3 : Mux  Inputs=5
  PIP_rise_perc : Constant  Value=PIP_rise_perc  OutDataTypeStr=single
  Product : Product
  Product1 : Product
  Product2 : Product  Inputs=**/*
  a0 : Fcn  Expr=u(3)+u(2)+u(1)-8
  a1 : Fcn  Expr=-u(3)+u(2)+3*u(1)+24
  a2 : Fcn  Expr=-u(3)-u(2)+3*u(1)-24
  a3 : Fcn  Expr=u(3)-u(2)+u(1)+8
  b0_3 : Fcn  Expr=u(1)
  b1_2 : Fcn  Expr=3*u(1)
  fun : Fcn  Expr=(u(3)-u(1)) / (u(2)*(u(3)+u(4)+u(5)) + u(3)*(2*u(2)+u(1)))
  fun1 : Fcn  Expr=u/(u+1)
  Num : Outport
  Den : Outport  Port=2
  x0_Gain : Outport  Port=3
  wires:
  Gain/1 -> Mux/3, Product/1, Math Function/1  "PC_IST"
  Math Function/1 -> Product/2, Mux/2
  Mux/1 -> Divide/2
  Constant/1 -> Divide/1
  Divide/1 -> Product1/1  "abc"
  Product/1 -> Mux/1
  Constant1/1 -> Product1/2
  Product1/1 -> b1_2/1, b0_3/1, a3/1, a2/1, a1/1, a0/1  "pnm"
  b0_3/1 -> Divide1/1
  b1_2/1 -> Divide2/1
  a0/1 -> Divide5/2, Divide4/2, Divide3/2, Divide2/2, Divide1/2
  a1/1 -> Divide3/1
  Mux1/1 -> Num/1
  Divide1/1 -> Mux3/1, Mux1/4, Mux1/1
  Divide2/1 -> Mux3/2, Mux1/2, Mux1/3
  Mux2/1 -> Den/1
  Constant2/1 -> Mux2/1
  Mux3/1 -> fun/1
  fun/1 -> x0_Gain/1
  a2/1 -> Divide4/1
  a3/1 -> Divide5/1
  Divide3/1 -> Mux3/3, Mux2/2
  Divide4/1 -> Mux3/4, Mux2/3
  Divide5/1 -> Mux3/5, Mux2/4
  IE_ratio/1 -> fun1/1
  Product2/1 -> Gain/1
  PIP_rise_perc/1 -> Product2/1
  Constant 1/1 -> Product2/2
  BPM/1 -> Product2/3
  fun1/1 -> Product2/4

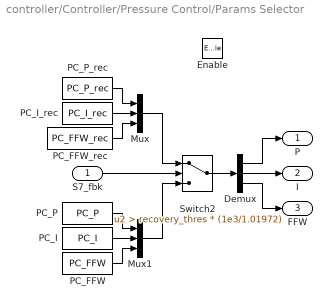
== system controller/Controller/Pressure Control/Params Selector ==
  S7_fbk : Inport
  Enable : EnablePort  StatesWhenEnabling=reset
  Demux : Demux  Outputs=3
  Mux : Mux  Inputs=3
  Mux1 : Mux  Inputs=3
  PC_FFW : Constant  Value=PC_FFW  OutDataTypeStr=single
  PC_FFW_rec : Constant  Value=PC_FFW_rec  OutDataTypeStr=single
  PC_I : Constant  Value=PC_I  OutDataTypeStr=single
  PC_I_rec : Constant  Value=PC_I_rec  OutDataTypeStr=single
  PC_P : Constant  Value=PC_P  OutDataTypeStr=single
  PC_P_rec : Constant  Value=PC_P_rec  OutDataTypeStr=single
  Switch2 : Switch  Criteria=u2 > Threshold  Threshold=recovery_thres * (1e3/1.01972)
  P : Outport  InitialOutput=PC_P
  I : Outport  Port=2  InitialOutput=PC_I
  FFW : Outport  Port=3  InitialOutput=PC_FFW
  wires:
  Mux/1 -> Switch2/1
  Mux1/1 -> Switch2/3
  S7_fbk/1 -> Switch2/2
  Switch2/1 -> Demux/1
  Demux/2 -> I/1
  Demux/1 -> P/1
  Demux/3 -> FFW/1
  PC_I_rec/1 -> Mux/2
  PC_P_rec/1 -> Mux/1
  PC_FFW_rec/1 -> Mux/3
  PC_I/1 -> Mux1/2
  PC_P/1 -> Mux1/1
  PC_FFW/1 -> Mux1/3

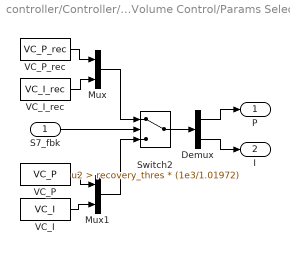
== system controller/Controller/Volume Control/Params Selector ==
  S7_fbk : Inport
  Demux : Demux  Outputs=2
  Mux : Mux  Inputs=2
  Mux1 : Mux  Inputs=2
  Switch2 : Switch  Criteria=u2 > Threshold  Threshold=recovery_thres * (1e3/1.01972)
  VC_I : Constant  Value=VC_I  OutDataTypeStr=single
  VC_I_rec : Constant  Value=VC_I_rec  OutDataTypeStr=single
  VC_P : Constant  Value=VC_P  OutDataTypeStr=single
  VC_P_rec : Constant  Value=VC_P_rec  OutDataTypeStr=single
  P : Outport  InitialOutput=PC_P
  I : Outport  Port=2  InitialOutput=PC_I
  wires:
  Mux/1 -> Switch2/1
  Mux1/1 -> Switch2/3
  S7_fbk/1 -> Switch2/2
  Switch2/1 -> Demux/1
  Demux/2 -> I/1
  Demux/1 -> P/1
  VC_I_rec/1 -> Mux/2
  VC_P_rec/1 -> Mux/1
  VC_I/1 -> Mux1/2
  VC_P/1 -> Mux1/1

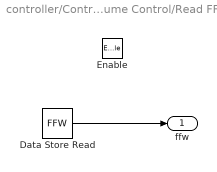
== system controller/Controller/Volume Control/Read FFW ==
  Enable : EnablePort
  Data Store Read : DataStoreRead  DataStoreName=FFW
  ffw : Outport  OutputWhenDisabled=reset  InitialOutput=0
  wires:
  Data Store Read/1 -> ffw/1

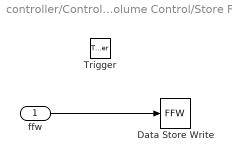
== system controller/Controller/Volume Control/Store FFW ==
  ffw : Inport
  Trigger : TriggerPort  TriggerType=falling  VariantControl=Variant  PortDimensions=1
  Data Store Write : DataStoreWrite  DataStoreName=FFW
  wires:
  ffw/1 -> Data Store Write/1

== stateflow chart controller/Controller/TD Max ==
  settings: executeAtInitialization=1
  state IDLE
    entry:
    TD_max = realmax('single');
  state COMPUTE_MAX
    entry:
    tmp_max = TD;
    during:
    tmp_max = max(tmp_max, TD);
  (default) -> IDLE
  IDLE -> COMPUTE_MAX : [compute]
  COMPUTE_MAX -> IDLE [order 1] : [~compute]
  COMPUTE_MAX -> COMPUTE_MAX [order 2] : after(2*(60/BPM), sec)/{TD_max = tmp_max;}
  data: BPM input single size=1; compute input boolean size=1; TD input single size=1; TD_max output single size=1; tmp_max local single size=1

== stateflow chart controller/Controller/Pulse Generator ==
  settings: executeAtInitialization=1
  state TRIGGER_WAIT
    entry:
    pulse = 0;
  state TRIGGER_INSPIRATION
    entry:
    pulse = 1;
  state INSPIRATION
    entry:
    pulse = 1;
  state EXPIRATION
    entry:
    pulse = 0;
  TRIGGER_WAIT -> INSPIRATION [order 2] : [~enable_trigger]
  INSPIRATION -> TRIGGER_WAIT [order 3] : [enable_trigger]
  TRIGGER_INSPIRATION -> TRIGGER_WAIT [order 1] : after(IE_ratio/(IE_ratio+1) * (60/BPM), sec)
  TRIGGER_WAIT -> TRIGGER_INSPIRATION [order 1] : [trigger]
  (default) -> INSPIRATION
  INSPIRATION -> INSPIRATION [order 1] : [hasChanged(control_mode)]
  TRIGGER_INSPIRATION -> INSPIRATION [order 2] : [~enable_trigger]
  INSPIRATION -> EXPIRATION [order 2] : after(IE_ratio/(IE_ratio+1) * (60/BPM), sec)
  EXPIRATION -> INSPIRATION [order 1] : [hasChanged(control_mode)]
  EXPIRATION -> INSPIRATION [order 2] : after(1/(IE_ratio+1) * (60/BPM), sec)
  data: BPM input single size=1; IE_ratio input single size=1; pulse output single size=1; control_mode input size=1; enable_trigger input boolean size=1; trigger input boolean size=1
